simulink model "inv_rot_pen_analytical_sim"  (R2024a)
settings: Solver=VariableStepAuto  StartTime=0.0  StopTime=10.0  RelTol=1e-3
values from neighbouring files (symbols this model uses):
  theta0 = [0; pi+pi/9]    [inv_rot_pen_ini.m]
settings Model: Creator=pichim  LastModifiedBy=pichim

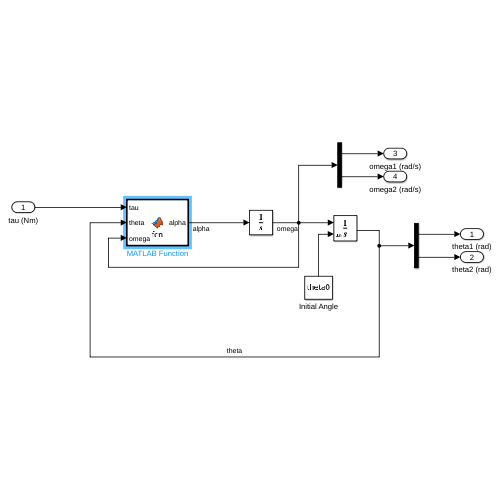
[thumbnail: Simulink's stored preview of the top-level diagram]
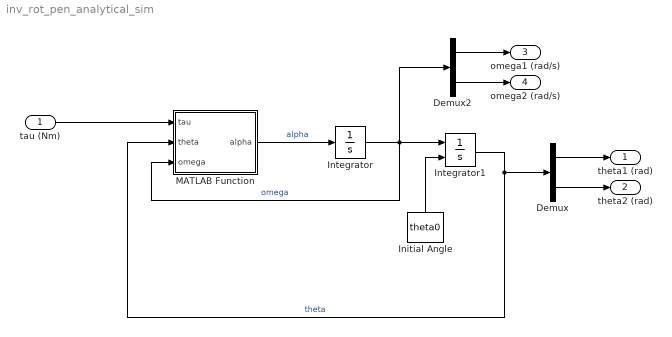
== system inv_rot_pen_analytical_sim ==
  tau (Nm) : Inport
  Demux : Demux  Outputs=2
  Demux2 : Demux  Outputs=2
  Initial Angle : Constant  Value=theta0
  Integrator : Integrator
  Integrator1 : Integrator  InitialConditionSource=external  InitialCondition=[0.1;0]
  MATLAB Function : MATLAB Function  TreatAsAtomicUnit=on
  theta1 (rad) : Outport
  theta2 (rad) : Outport  Port=2
  omega1 (rad/s) : Outport  Port=3
  omega2 (rad/s) : Outport  Port=4
  wires:
  tau (Nm)/1 -> MATLAB Function/1(tau)
  Initial Angle/1 -> Integrator1/2
  Demux/1 -> theta1 (rad)/1
  Demux2/1 -> omega1 (rad/s)/1
  Integrator/1 -> MATLAB Function/3(omega), Demux2/1, Integrator1/1  "omega"
  Demux2/2 -> omega2 (rad/s)/1
  Demux/2 -> theta2 (rad)/1
  Integrator1/1 -> MATLAB Function/2(theta), Demux/1  "theta"
  MATLAB Function/1(alpha) -> Integrator/1  "alpha"

== matlab function inv_rot_pen_analytical_sim/MATLAB Function ==
  data: tau input size=1; alpha output size=[2,1]; theta input size=[2,1]; omega input size=[2,1]; param parameter
function alpha = fcn(tau, theta, omega, param)

    % M(q) * qdd + C(q,qdot) * qdot + G(q) + D * qdot = tau
    [M, C, G, D] = calculate_dynamics_furuta(theta, omega, param);
    alpha = M \ ( [tau; 0] - (C + D) * omega - G );

end
